simulink model "observateur"  (R2025b)
settings: Solver=FixedStepAuto  StartTime=0.0  StopTime=inf  RelTol=1e-3  EnableMultiTasking=on
values from neighbouring files (symbols this model uses):
  Aobs = Ad-Lo*Cd    [AncienTest.m]
  Bobs = [Bd Lo]    [AncienTest.m]
  Cobs = eye(2)    [AncienTest.m]
  Dobs = zeros(2)    [AncienTest.m]
  K_corr = acker(Ad,Bd,poles_souhaites)    [AncienTest.m]    (also in Test.m)
  S_corr = inv(Cd*inv(eye(2)-Ad+Bd*K_corr)*Bd)    [AncienTest.m]    (also in Test.m)
  Te = 1/100    (= 0.01)    [AncienTest.m]    (also in Test.m)
libraries: legoev3lib x2
settings Model: ExtModeTrigDuration=2  Creator=carol  LastModifiedBy=carol
settings SolverCC: PositivePriorityOrder=on
settings OptimizationCC: DefaultParameterBehavior=Inlined  EnhancedBackFolding=on  PassReuseOutputArgsAs=Individual arguments  ZeroExternalMemoryAtStartup=off  ZeroInternalMemoryAtStartup=off  MaxStackSize=64  OptimizeBlockOrder=speed  DifferentSizesBufferReuse=on  OptimizationCustomize=off  EfficientTunableParamExpr=on
settings DebuggingCC: ParameterTunabilityLossMsg=error
settings HardwareCC: ProdBitPerPointer=32.0  ProdBitPerSizeT=32.0  ProdBitPerPtrDiffT=32.0  ProdLargestAtomicInteger=Long  ProdWordSize=32.0  ProdHWDeviceType=ARM Compatible->ARM 9  UseEmbeddedCoderFeatures=off  UseSimulinkCoderFeatures=off
settings SFSimCC: MATLABDynamicMemAlloc=off
settings RTWCC: SystemTargetFile=ert.tlc  HardwareBoard=LEGO MINDSTORMS EV3  TLCOptions="-aInlineSetEventsForThisBaseRateFcn=TLC_FALSE -aSuppressMultiTaskScheduler=TLC_FALSE  -aRateBasedStepFcn=0"  TemplateMakefile=ert_default_tmf  Toolchain=Sourcery G++ Lite v2009q3  Description=Embedded Coder
settings CodeAppCC: ForceParamTrailComments=on  IgnoreCustomStorageClasses=off  OperatorAnnotations=on  SimulinkDataObjDesc=on  SFDataObjDesc=on  InsertBlockDesc=on
settings ERTTargetCC: ExtModeTransport=2.0  ExtModeStaticAlloc=on  ExtModeMexFile=ext_xcp  ExtModeIntrfLevel=Level2 - Open  SupportContinuousTime=on  SupportNonInlinedSFcns=on  SupportVariableSizeSignals=on

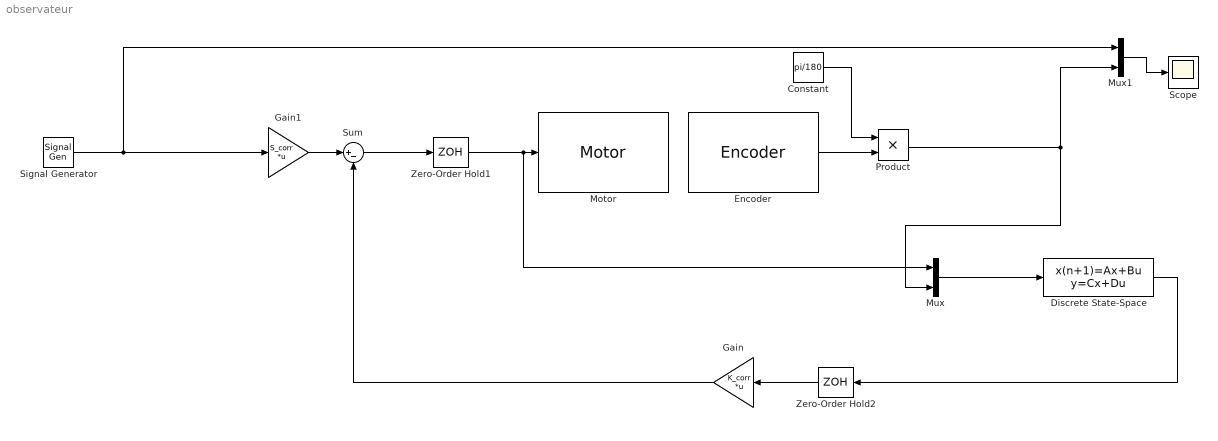
== system observateur ==
  Constant : Constant  Value=pi/180
  Discrete State-Space : DiscreteStateSpace  A=Aobs  B=Bobs  C=Cobs  D=Dobs  SampleTime=Te
  Encoder : legoev3lib/Encoder  portNumber=D  opMode=Reset by external signal  sampleTime=Te
  Gain : Gain  Gain=K_corr  Multiplication=Matrix(K*u)
  Gain1 : Gain  Gain=S_corr  Multiplication=Matrix(K*u)
  Motor : legoev3lib/Motor  sportNumber=D  sstopAction=Brake
  Mux : Mux  Inputs=2
  Mux1 : Mux  Inputs=2
  Product : Product
  Scope : Scope
      settings: ActiveDisplayYMinimum=-30.370979428831127  ActiveDisplayYMaximum=33.700651401798282
  Signal Generator : SignalGenerator  WaveForm=square  Frequency=0.1
  Sum : Sum  Inputs=|+-
  Zero-Order Hold1 : ZeroOrderHold  SampleTime=Te
  Zero-Order Hold2 : ZeroOrderHold  SampleTime=Te
  wires:
  Encoder/1 -> Product/2
  Zero-Order Hold1/1 -> Mux/1, Motor/1
  Signal Generator/1 -> Mux1/1, Gain1/1
  Sum/1 -> Zero-Order Hold1/1
  Gain1/1 -> Sum/1
  Gain/1 -> Sum/2
  Product/1 -> Mux1/2, Mux/2
  Constant/1 -> Product/1
  Zero-Order Hold2/1 -> Gain/1
  Mux1/1 -> Scope/1
  Mux/1 -> Discrete State-Space/1
  Discrete State-Space/1 -> Zero-Order Hold2/1
